simulink model "Verifica_LQG_05062026"  (R2025b)
settings: Solver=ode4  StartTime=0.0  StopTime=1e3  FixedStep=0.01  RelTol=1e-3
undefined symbols (not defined in the file): A, A_kalman, B, B_kalman, C_kalman, C_LQR, D, D_kalman, K_LQR_i, K_LQR_x, r_lqr, x0_LQR
libraries: simulink x2
settings Model: Creator=salvo  LastModifiedBy=salvo

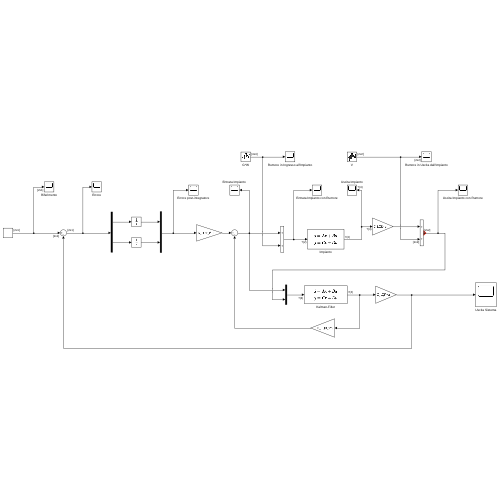
[thumbnail: Simulink's stored preview of the top-level diagram]
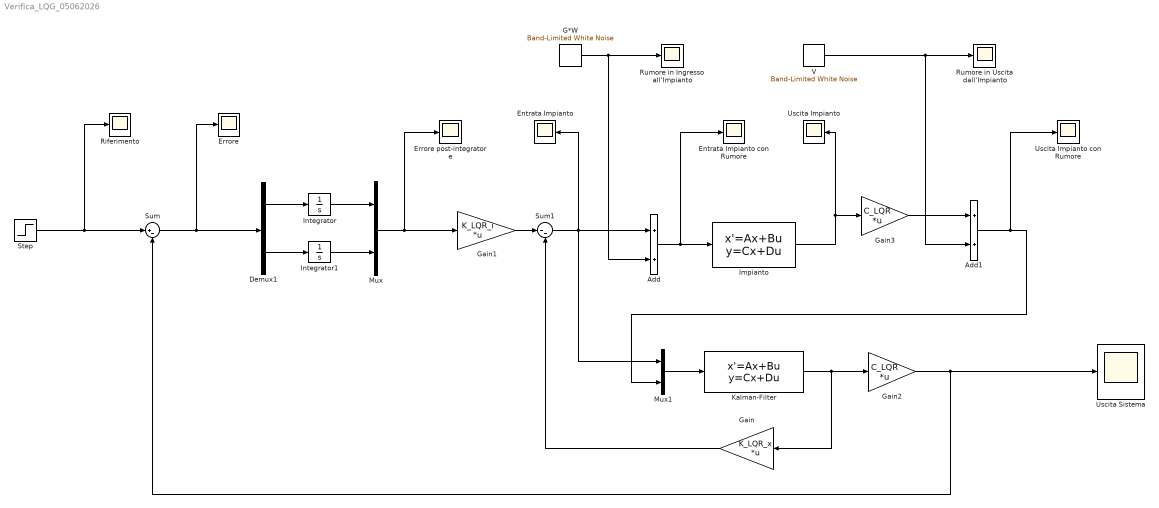
== system Verifica_LQG_05062026 ==
  Add : Sum
  Add1 : Sum
  Demux1 : Demux  Outputs=2
  "Entrata Impianto " : Scope
      settings: ActiveDisplayYMinimum=-12.425296545866741  ActiveDisplayYMaximum=13.733770865887159  DataLoggingVariableName=ScopeData5
  Entrata Impianto con Rumore : Scope
      settings: DataLoggingVariableName=ScopeData6
  Errore : Scope
      settings: ActiveDisplayYMinimum=-0.29418197151740361  ActiveDisplayYMaximum=0.99885841903562977  DataLoggingVariableName=ScopeData3
  Errore post-integratore : Scope
      settings: ActiveDisplayYMinimum=0.22349407279263428  ActiveDisplayYMaximum=0.582778285880051  DataLoggingVariableName=ScopeData4
  G*W : simulink/Sources/Band-Limited White Noise  Cov=0.1*eye(4)  Ts=0.1  seed=[23341]
  Gain : Gain  Gain=K_LQR_x  Multiplication=Matrix(K*u)
  Gain1 : Gain  Gain=K_LQR_i  Multiplication=Matrix(K*u)
  Gain2 : Gain  Gain=C_LQR  Multiplication=Matrix(K*u)
  Gain3 : Gain  Gain=C_LQR  Multiplication=Matrix(K*u)
  Impianto : StateSpace  A=A  B=B  C=eye(4)  D=[D;zeros(2,2)]  InitialCondition=x0_LQR
  Integrator : Integrator
  Integrator1 : Integrator
  Kalman-Filter : StateSpace  A=A_kalman  B=B_kalman  C=C_kalman  D=D_kalman  InitialCondition=0
  Mux : Mux  Inputs=2
  Mux1 : Mux  Inputs=2
  Riferimento : Scope
      settings: ActiveDisplayYMinimum=-0.00055584265063463034  ActiveDisplayYMaximum=0.22392619810213177  DataLoggingVariableName=ScopeData2
  Rumore in Ingresso all'Impianto : Scope
  Rumore in Uscita dall'Impianto : Scope
      settings: DataLoggingVariableName=ScopeData7
  Step : Step  After=r_lqr  SampleTime=0  VectorParams1D=off
  Sum : Sum  Inputs=|+-
  Sum1 : Sum  Inputs=|--
  Uscita Impianto : Scope
      settings: ActiveDisplayYMinimum=-60.802742744001982  ActiveDisplayYMaximum=58.710565995268688
  Uscita Impianto con Rumore : Scope
      settings: DataLoggingVariableName=ScopeData8
  Uscita Sistema : Scope
      settings: DataLoggingVariableName=ScopeData9
  V : simulink/Sources/Band-Limited White Noise  Cov=0.001*eye(2)  Ts=0.1  seed=[23341]
  wires:
  Gain1/1 -> Sum1/1
  Demux1/2 -> Integrator1/1
  Gain/1 -> Sum1/2
  Demux1/1 -> Integrator/1
  Integrator1/1 -> Mux/2
  Sum/1 -> Errore/1, Demux1/1
  Mux/1 -> Gain1/1, Errore post-integratore/1
  Integrator/1 -> Mux/1
  Impianto/1 -> Uscita Impianto/1, Gain3/1
  Sum1/1 -> Mux1/1, "Entrata Impianto "/1, Add/1
  Step/1 -> Riferimento/1, Sum/1
  Add/1 -> Impianto/1, Entrata Impianto con Rumore/1
  G*W/1 -> Add/2, Rumore in Ingresso all'Impianto/1
  V/1 -> Add1/2, Rumore in Uscita dall'Impianto/1
  Mux1/1 -> Kalman-Filter/1
  Add1/1 -> Uscita Impianto con Rumore/1, Mux1/2
  Kalman-Filter/1 -> Gain/1, Gain2/1
  Gain2/1 -> Sum/2, Uscita Sistema/1
  Gain3/1 -> Add1/1
